simulink model "ac3_example_MMCT"  (R2023a)
settings: Solver=FixedStepDiscrete  StartTime=0.0  StopTime=3  FixedStep=Ts  RelTol=1e-3  EnableMultiTasking=on
PreLoadFcn:
  | Ts = 2e-6;
undefined symbols (not defined in the file): DiscIntNeverNeededParam
libraries: simulink_extras x7, spsCurrentMeasurementLib x3, spsVoltageMeasurementLib x3, spsDrivesPrivateModels x2, spsStairGeneratorLib x2, spsThreePhaseSourceLib x1, spsDrivesDcBusModel x1, spsSpaceVectorModulatorLib x1, eeAdaptiveController x1, slctrlblks x1, simulink x1, slpidlib x1
(part 1 of 3)
settings Model: Creator=The MathWorks, Inc.  LastModifiedBy=13372
settings SolverCC: AlgebraicLoopSolver=TrustRegion
settings DataIOCC: LimitDataPoints=on  SaveFormat=Array  SaveOutput=off  SignalLogging=off  SaveTime=off  ReturnWorkspaceOutputs=off  SignalLoggingName=sigsOut
settings OptimizationCC: ExpressionDepthLimit=2147483647  InitFltsAndDblsToZero=on  LifeSpan=inf
settings DebuggingCC: UnderspecifiedInitializationDetection=Classic  MergeDetectMultiDrivingBlocksExec=none  CheckExecutionContextPreStartOutputMsg=on  SignalResolutionControl=TryResolveAllWithWarning  MultiTaskDSMMsg=warning  MultiTaskCondExecSysMsg=none  FcnCallInpInsideContextMsg=warning  UnconnectedInputMsg=warning  UnconnectedOutputMsg=warning  UnconnectedLineMsg=warning  StateNameClashWarn=warning  SFUnexpectedBacktrackingDiag=warning  SFNoUnconditionalDefaultTransitionDiag=warning  SFExecutionAtInitializationDiag=none  ArithmeticOperatorsInVariantConditions=warning
settings HardwareCC: ProdBitPerPointer=32  ProdBitPerSizeT=32  ProdBitPerPtrDiffT=32  ProdLargestAtomicFloat=None  ProdIntDivRoundTo=Undefined  ProdEndianess=Unspecified  ProdWordSize=32  ProdHWDeviceType=32-bit Generic  TargetUnknown=on
settings ModelReferenceCC: EnableRefExpFcnMdlSchedulingChecks=on  PropagateSignalLabelsOutOfModel=off
settings SFSimCC: SimUseLocalCustomCode=off  CustomCodeUndefinedFunction=UseInterfaceOnly
settings RTWCC: RTWUseLocalCustomCode=off
settings CodeAppCC: StateflowObjectComments=on
settings GRTTargetCC: TargetLangStandard=C89/C90 (ANSI)  CombineOutputUpdateFcns=off  GRTInterface=on
settings ConfigComp: CovMetricSettings=dw  CovSaveCumulativeToWorkspaceVar=on  CovSaveSingleToWorkspaceVar=on  CovExternalEMLEnable=off  CovSFcnEnable=off
settings SimscapeCC: SimscapeNormalizeSystem=off

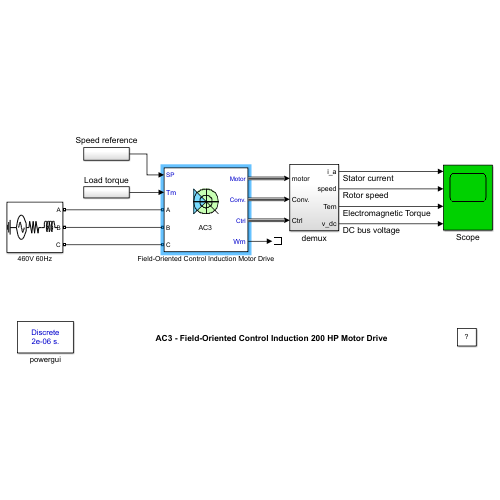
[thumbnail: Simulink's stored preview of the top-level diagram]
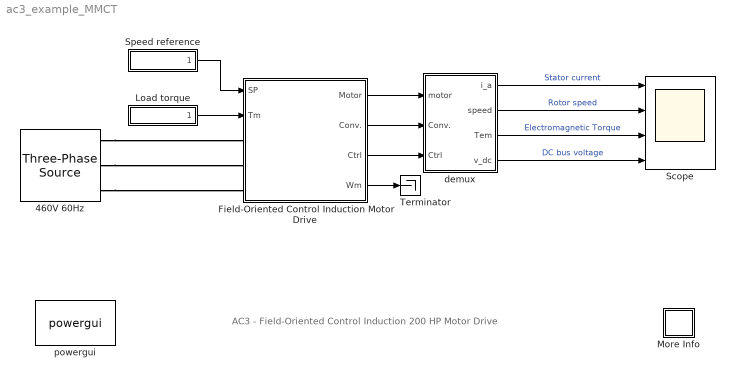
== system ac3_example_MMCT ==
  note: AC3 - Field-Oriented Control Induction 200 HP Motor Drive
  460V 60Hz : spsThreePhaseSourceLib/Three-Phase Source  InternalConnection=Yg  VoltagePhases=off  Voltage=460  PhaseAngle=0  Voltage_phases=[25e3 25e3 25e3]/sqrt(3)  PhaseAngles_phases=[0 -120 +120]  Frequency=60  NonIdealSource=on  SpecifyImpedance=off  Resistance=0.02  Inductance=0.05e-3  ShortCircuitLevel=100e6  BaseVoltage=25e3  XRratio=7  BusType=swing  Pref=0  Qref=0  Prefabc=[10e3, 10e3, 10e3]  Qrefabc=[0, 0, 0]  Qmin=-inf  Qmax=inf
  Field-Oriented Control Induction Motor Drive : Subsystem  AncestorBlock=electricdrivelib/AC drives/Field-Oriented Control Induction Motor Drive  DialogController=POWERSYS.PowerSysDialog  LoadFcn=|  mask(Field-Oriented Control Induction Motor Drive){ReferenceFrame=Rotor, IterativeDiscreteModel=Trapezoidal non iterative, Pn=149.2e3, Vn=460, fn=60, Rs=14.85e-3, Lls=0.3027e-3, Lms=10.46e-3, Rr=9.295e-3, Llr=0.3027e-3, ia=0, pha=0, ib=0, phb=0, ic=0, phc=0, J=3.1, Friction=0.08, p=2, slip=1, thdeg=0, Rsnb_rec=10e3, Csnb_rec=20e-9, Ron_rec=1e-3, Vf_rec=1.3, cap_bus=7500e-6, Rbrake=8, fbrake=4000, activationVoltage=700, shutdownVoltage=660, sourceFrequency=60, deviceType=IGBT / Diodes, Ron_inv=1e-3, Vf_inv=0.8, Vfd_inv=0.8, Tf=1e-6, Tt=2e-6, Tf_GTO=10e-6, Tt_GTO=20e-6, Rsnb_inv=5e3, Csnb_inv=inf, regulationType=Speed regulation, Acc=900, Dec=-900, kp_sc=300, ki_sc=2000, fc_sc=1000, Tsc=100e-6, Tmin=-1200, Tmax=1200, in_flux=0.73, nf=0.73, kp_fc=100, ki_fc=30, freqc_fc=16, fluxmin=-2, fluxmax=2, modulationType=SVM, h=10, kp_Id=5, ki_Id=100, kp_Iq=5, ki_Iq=100, fc_bus=50, car_freq=20000, freq_max=20000, Tvect=20e-6, zeta=0.9, Trd=0.1, bwRatio=30, kp_estimator=5000, ki_estimator=50, upperLimit=500, lowerLimit=-500, Testimator=2e-06, baseSampleTime=2e-06, outputBusMode=Multiple output buses, busLabels=off, sensorless=off, MechanicalLoad=Torque Tm, modelDetailLevel=Detailed, driveType=AC3, AverageValue=off}
      | if ~isempty(get_param(gcb,'UserData')) 
      |       UserDataToSimulinkMask(gcbh,get_param(gcb,'driveType'));  
      |       set_param(gcb, 'UserData',[]);
      |       set_param(gcb,'UserDataPersistent','off');
      | end 
      | 
      | if strcmp(get_param(gcb,'AverageValue'),'on')
      |     set_param(gcb,'modelDetailLevel','Average');
      | end
      mask prompts: ReferenceFrame "Reference frame:"; IterativeDiscreteModel "Discrete solver model:"; Pn "Power (VA):"; Vn "Voltage (Vrms):"; fn "Frequency (Hz):"; Rs "Resistance (ohm):"; Lls "Leakage inductance (H):"; Lms "Mutual inductance (H):"; Rr "Resistance (ohms):"; Llr "Leakage inductance (H):"; ia "Ia_Magnitude (A)"; pha "Ia_Phase (deg)"; ib "Ib_Magnitude (A)"; phb "Ib_Phase (deg)"; ic "Ic_Magnitude (A)"; phc "Ic_Phase (deg)"; J "Inertia (kg.m^2):"; Friction "Friction factor (N.m.s):"; p "Pole pairs:"; thdeg "Angle (deg):"; Rsnb_rec "Resistance (ohm):"; Csnb_rec "Capacitance (F):"; Ron_rec "On-state resistance (ohm):"; Vf_rec "Forward voltage (V):"; cap_bus "Capacitance (F):"; Rbrake "Resistance (ohm):"; fbrake "Chopper frequency (Hz):"; activationVoltage "Activation voltage (V):"; shutdownVoltage "Shutdown voltage (V):"; sourceFrequency "Source frequency (Hz):"; deviceType "Device type:"; Ron_inv "On-state resistance (ohm):"; Vf_inv "Main device:"; Vfd_inv "Diode:"; Tf "Fall time (s):"; Tt "Tail time (s):"; Tf_GTO "Fall time (s):"; Tt_GTO "Tail time (s):"; Rsnb_inv "Resistance (ohm):"; Csnb_inv "Capacitance (F):"; regulationType "Regulation type:"; Acc "Acceleration:"; Dec "Deceleration:"; kp_sc "Proportional gain:"; ki_sc "Integral gain:"; fc_sc "Speed cutoff frequency (Hz):"; Tsc "Speed controller sampling time (s):"; Tmin "Negative:"; Tmax "Positive:"; in_flux "Initial:"; nf "Nominal:"; kp_fc "Proportional gain:"; ki_fc "Integral gain:"; freqc_fc "Low-pass filter cutoff frequency (Hz):"; fluxmin "Negative:"; fluxmax "Positive:"; modulationType "Modulation type:"; h "Current controller hysteresis bandwidth (A):"; kp_Id "Proportional gain:"; ki_Id "Integral gain:"; kp_Iq "Proportional gain:"; ki_Iq "Integral gain:"; fc_bus "DC bus voltage sensor cutoff frequency (Hz):"; car_freq "SVM switching frequency (Hz):"; freq_max "Maximum  switching frequency (Hz):"; Tvect "Controller sampling time (s):"; zeta "Desired damping [zeta] :"; Trd "Desired response time @ 5% [Trd (sec)] :"; bwRatio "Bandwidth ratio (InnerLoop/SpeedLoop) :"; kp_estimator "Proportional gain:"; ki_estimator "Integral gain:"; upperLimit "Upper:"; lowerLimit "Lower:"; Testimator "Controller Sample Time"; baseSampleTime "Base sample time:"; outputBusMode "Output bus mode:"; busLabels "Use bus labels"; sensorless "Set sensorless"; MechanicalLoad "Mechanical input:"; modelDetailLevel "Model detail level:"; driveType "Drive type:"; AverageValue "Average value model"
      mask help: Implements a standard vector or rotor field-oriented control drive for induction motors.
      mask init:
      | [X1,X1m,X2,X2m,X3,X4,Y1,Y1m,Y2,Y2m,Y3,Y4,color1,color2,INp,OUTp,machineType,baseSampleTime] = spsDrivesMaskInit(gcb,driveType,AverageValue);
      settings: OpenFcn=sps_rtmsupport('OpenFcn',gcbh)
      settings: LibrarySourceBlock=|
      | electricdrivelib/AC drives/Field-Oriented Control
      | Induction Motor Drive
      mask Help: helpview(psbhelp)
      mask TypeOptions ReferenceFrame: Rotor | Stationary | Synchronous
      mask Callback ReferenceFrame: set_param([gcb '/Induction machine'],'ReferenceFrame',get_param(gcb,'ReferenceFrame'));
      mask TypeOptions IterativeDiscreteModel: Forward Euler | Trapezoidal non iterative
      mask Callback IterativeDiscreteModel: %set_param(gcb,'IterativeDiscreteModel',get_param([gcb '/Induction machine'],'IterativeModel'));
      mask Callback Pn: %set(gcf,'Color',[0.3,0.7,0.1])
      mask TypeOptions deviceType: GTO / Diodes | MOSFET / Diodes | IGBT / Diodes
      mask Callback deviceType:
      | set_param([gcb,'/Three-phase Inverter'],'Device',get_param(gcb,'deviceType'));
      | spsDrivesMaskController(gcb,get_param(gcb,'driveType'),get_param(gcb,'averageValue'));
      mask TypeOptions regulationType: Speed regulation | Torque regulation
      mask Callback regulationType:
      | set_param([gcb '/Speed Controller'],'SwK',get_param(gcb,'regulationType'));
      | spsDrivesMaskController(gcb,get_param(gcb,'driveType'),get_param(gcb,'averageValue'));
      mask TypeOptions modulationType: Hysteresis | SVM
      mask Callback modulationType:
      | spsDrivesMaskController(gcb,get_param(gcb,'driveType'),get_param(gcb,'averageValue'));
      | %spsDrivesSetModulation(gcb,get_param(gcb,'driveType'),get_param(gcb,'averageValue'));
      mask TypeOptions outputBusMode: Multiple output buses | Single output bus
      mask Callback sensorless:
      | %spsDrivesSetSensorless(gcb,get_param(gcb,'driveType'),get_param(gcb,'sensorless'));
      | spsDrivesMaskController(gcb,get_param(gcb,'driveType'),get_param(gcb,'averageValue'));
      | %spsDrivesSetSensorless(gcb,get_param(gcb,'driveType'),get_param(gcb,'sensorless'));
      | %spsDrivesMaskController(gcb,get_param(gcb,'driveType'),get_param(gcb,'averageValue'));
      mask TypeOptions MechanicalLoad: Torque Tm | Speed w | Mechanical rotational port
      mask Callback MechanicalLoad: spsDrivesMaskController(gcb,get_param(gcb,'driveType'),get_param(gcb,'averageValue'));
      mask TypeOptions modelDetailLevel: Detailed | Average
      mask Callback modelDetailLevel:
      | if strcmp(get_param(gcb,'modelDetailLevel'),'Average')
      |    set_param(gcb,'AverageValue','on');
      |    spsDrivesMaskController(gcb,get_param(gcb,'driveType'),1);
      | else
      |    set_param(gcb,'AverageValue','off');
      |    spsDrivesMaskController(gcb,get_param(gcb,'driveType'),0);
      | end
      mask TypeOptions driveType: AC3
      mask DialogControl Container7 Prompt: Asynchronous Machine
      mask DialogControl Container22 Prompt: Electrical parameters
      mask DialogControl Container24 Prompt: Nominal values
      mask DialogControl Container27 Prompt: Equivalent circuit values
      mask DialogControl Container25 Prompt: Main winding stator
      mask DialogControl Container21 Prompt: Main winding rotor
      mask DialogControl Container34 Prompt: Initial currents
      mask DialogControl Container23 Prompt: Mechanical parameters
      mask DialogControl Container36 Prompt: Initial  values
      mask DialogControl Container10 Prompt: Converters and DC bus
      mask DialogControl Container28 Prompt: Rectifier
      mask DialogControl Container39 Prompt: Snubbers
      mask DialogControl Container40 Prompt: Diodes
      mask DialogControl Container30 Prompt: DC bus
      mask DialogControl Container31 Prompt: Braking chopper
      mask DialogControl Container32 Prompt: Inverter
      mask DialogControl Container41 Prompt: Switches
      mask DialogControl Forwardvoltages Prompt: Forward voltages (V)
      mask DialogControl Turnoff Prompt: Turn-off characteristics
      mask DialogControl InvSnubbers Prompt: Snubbers
      mask DialogControl Container12 Prompt: Controller
      mask DialogControl Control5 Prompt: Schematic
      mask DialogControl Control5 Callback:
      | openfig('ac3.fig','invisible');
      | movegui(gcf,'northwest');
      | set(gcf,'Visible','on');
      mask DialogControl SpeedController Prompt: Speed controller
      mask DialogControl Speedramp Prompt: Speed ramps (rpm/s)
      mask DialogControl PIregulator Prompt: PI regulator
      mask DialogControl Container46 Prompt: Torque output limits (N.m)
      mask DialogControl Container37 Prompt: Machine flux (Wb)
      mask DialogControl FieldOrientedControl Prompt: Field oriented control
      mask DialogControl FluxRegulator Prompt: Flux controller
      mask DialogControl Container50 Prompt: Flux output limits (Wb)
      mask DialogControl d_axiscurrentregulator Prompt: d-axis current regulator
      mask DialogControl q_axiscurrentregulator Prompt: q-axis current regulator
      mask DialogControl autoTuningCtrlbtn Prompt: Hide Autotuning Control
      mask DialogControl autoTuningCtrlbtn Callback: spsDrivesAutotuningCbak(gcb,'visibility',get_param(gcb,'driveType'));
      mask DialogControl autoTuningContainer Prompt: Autotuning of PI loops
      mask DialogControl Control7 Prompt: Enter speed loop specifications
      mask DialogControl Calculate Prompt: Calculate PI regulators gains
      mask DialogControl Calculate Callback: spsDrivesAutotuningCbak(gcb,'PICalculator',get_param(gcb,'driveType'));
      mask DialogControl sensorlessTab Prompt: Sensorless
      mask DialogControl Container59 Prompt: Estimator controller parameters
      mask DialogControl Container61 Prompt: Output limits
      mask DialogControl Container56 Prompt: Parameters file options
      mask DialogControl Control3 Prompt: Load
      mask DialogControl Control3 Callback: loadValues(gcb,get_param(gcb,'driveType'));
      mask DialogControl Control4 Prompt: Save
      mask DialogControl Control4 Callback: saveValues(gcb,get_param(gcb,'driveType'));
      mask Display:
      | patch([X1 X1m],[Y1 Y1m],color1);
      | patch(X3,Y3,color2);
      | plot([X1 X1m X2 X2m X3 X4],[Y1 Y1m Y2 Y2m Y3 Y4]);
      | text(0.5,0.3,'AC3','HorizontalAlignment','center')
      | HaveSPSMec = (strcmp(MechanicalLoad,'Torque Tm') || strcmp(MechanicalLoad,'Speed w'));
      | color('blue');
      | if (HaveSPSMec==1 && strcmp(outputBusMode,'Multiple output buses'))
      |     port_label('input',2,INp)
      |     port_label('output',4,OUTp)
      | end
      | if (HaveSPSMec==1 && strcmp(outputBusMode,'Single output bus'))
      |     port_label('input',2,INp)
      |     port_label('output',2,OUTp)
      | end
  Load torque : Subsystem
  More Info : Subsystem
      settings: OpenFcn=showdemo(bdroot(gcb))
      mask Display: disp('?')
  Scope : Scope  NumInputPorts=4
  Speed reference : Subsystem
  Terminator : Terminator
  demux : Subsystem
  powergui : spspowerguiLib/powergui  Priority=2  SimulationMode=Discrete  SampleTime=Ts  frequency=60  Iterations=50  frequencyindice=60  Pbase=100e6  ErrMax=1e-4  UnitsV=kV  UnitsW=MW  buscounter=0  FunctionMessages=off  echomessages=off  EnableUseOfTLC=off  CurrentSourceSwitches=off  DisableSnubberDevices=off  DisableRonSwitches=off  DisableVfSwitches=off  DisplayEquations=off  AutomaticDiscreteSolvers=off  SolverType=Tustin/Backward Euler (TBE)  Interpol=off  ExternalGateDelay=off  methode=off  Ts=0  x0status=blocks  SPID=off  SwTol=0  HookPort=off  NonlinearTolerance=1e-4  nMaxIteration=100  ContinueOnMaxIteration=off  RestoreLinks=warning  ResistiveCurrentMeasurement=off  Frange=[0:2:500]  Ylog=off  Xlog=on  ShowGrid=off  save=off  variable=ZData  structure=simout  ZoomFFT=on  StartTime=0.05  cycles=7  DisplayStyle=1  fundamental=60  FreqAxis=off  MaxFrequency=20000  frequencyindicesteady=1  RmsSteady=1  display=off
  wires:
  demux/1(i_a) -> Scope/1  "Stator current"
  demux/2(speed) -> Scope/2  "Rotor speed"
  demux/3(Tem) -> Scope/3  "Electromagnetic Torque"
  demux/4(v_dc) -> Scope/4  "DC bus voltage"
  Field-Oriented Control Induction Motor Drive/1(Motor) -> demux/1(motor)
  Field-Oriented Control Induction Motor Drive/2(Conv.) -> demux/2(Conv.)
  Field-Oriented Control Induction Motor Drive/3(Ctrl) -> demux/3(Ctrl)
  Speed reference/1(" ") -> Field-Oriented Control Induction Motor Drive/1(SP)
  Load torque/1(" ") -> Field-Oriented Control Induction Motor Drive/2(Tm)
  Field-Oriented Control Induction Motor Drive/4(Wm) -> Terminator/1
  connections:
  460V 60Hz/RConn1 -- Field-Oriented Control Induction Motor Drive/LConn1
  460V 60Hz/RConn2 -- Field-Oriented Control Induction Motor Drive/LConn2
  460V 60Hz/RConn3 -- Field-Oriented Control Induction Motor Drive/LConn3

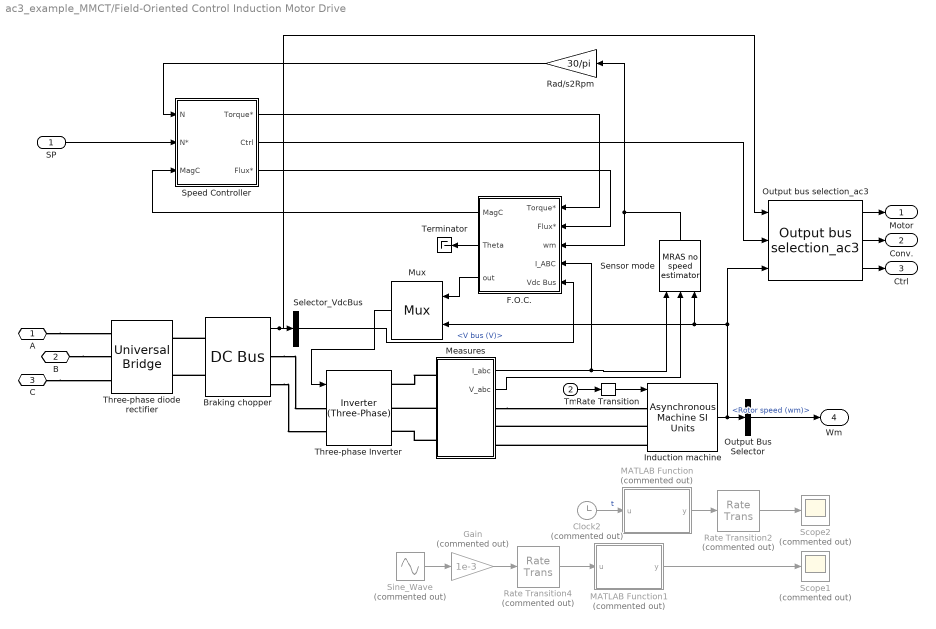
== system ac3_example_MMCT/Field-Oriented Control Induction Motor Drive ==
  SP : Inport
  Tm : Inport  Port=2
  Braking chopper : spsDrivesDcBusModel/DC Bus   busType=Capacitive (generic)  Ts=baseSampleTime  capacitance=cap_bus  inductance=0  Setx0=off  InitialVoltage=600  Rbrake=Rbrake  frequency=fbrake  activationVoltage=activationVoltage  shutdownVoltage=shutdownVoltage
  Clock2 : Clock  Commented=on
      settings: Decimation=3
  F.O.C. : Subsystem  AncestorBlock=spsFieldOrientedControllerLib/Field-Oriented Controller  DialogController=POWERSYS.PowerSysDialog  Variant=on  VariantControlMode=label  LabelModeActiveChoice=Detailed_SVM  mask(Field-Oriented Controller){detailLevel=Detailed, modulationType=SVM, kp=kp_fc, ki=ki_fc, fc=freqc_fc, csat=[fluxmin,fluxmax], Tvect=Tvect, Ts=baseSampleTime, h=h, freq_max=freq_max, fc_bus=fc_bus, car_freq=car_freq, kp_Id=kp_Id, ki_Id=ki_Id, kp_Iq=kp_Iq, ki_Iq=ki_Iq, Rr=Rr, Llr=Llr, Lm=Lms, p=p, in_flux=in_flux}
      mask prompts: detailLevel "Model detail level"; modulationType "Modulation type"; kp "Proportional gain"; ki "Integral gain"; fc "Low-pass filter cutoff frequency (Hz)"; csat "Controller output flux saturation (Wb) [Negative, Positive]"; Tvect "Vector control sampling time (s)"; Ts "Base sample time (s)"; h "Current regulator hysteresis bandwidth (A)"; freq_max "Maximum inverter frequency (Hz)"; fc_bus "DC bus voltage sensor cutoff frequency (Hz)"; car_freq "SVM switching frequency (Hz)"; kp_Id "Proportional gain"; ki_Id "Integral gain"; kp_Iq "Proportional gain"; ki_Iq "Integral gain"; Rr "Rotor resistance Rr' (Ohms)"; Llr "Rotor leakage inductance Llr' (H)"; Lm "Mutual inductance Lm (H)"; p "Pairs of poles"; in_flux "Initial flux (Wb)"
      mask help: This block implements a field oriented controller.
      mask init:
      | Lr=Lm+Llr;
      | [X1,X1m,X2,X2m,X3,X4,Y1,Y1m,Y2,Y2m,Y3,Y4,color1,color2]=spsdrivelogo;
      | block=gcb;
      | spsDrivesFieldOrientedControllercCbak(block);
      settings: AttributesFormatString=%<BlockChoice>  LibrarySourceBlock=spsFieldOrientedControllerLib/Field-Oriented Controller  OpenFcn=sps_rtmsupport('OpenFcn',gcbh)
      mask Help: helpview(psbhelp);
      mask TypeOptions detailLevel: Detailed | Average
      mask Callback detailLevel: spsDrivesFieldOrientedControllercCbak(gcb);
      mask TypeOptions modulationType: Hysteresis | SVM
      mask Callback modulationType: spsDrivesFieldOrientedControllercCbak(gcb);
      mask DialogControl ParameterTabVar01 Prompt: Controller
      mask DialogControl Container7 Prompt: Flux controller
      mask DialogControl daxis_gbox Prompt: d-axis current regulator
      mask DialogControl qaxis_gbox Prompt: q-axis current regulator
      mask DialogControl ParameterTabVar012 Prompt: Machine
      mask Display:
      | patch([X1 X1m],[Y1 Y1m],color1);
      | patch(X3,Y3,color2);
      | plot([X1 X1m X2 X2m X3 X4],[Y1 Y1m Y2 Y2m Y3 Y4]);
      | block=gcb;
      | detailLevel = get_param(block,'detailLevel');
      | color('blue');
      | switch detailLevel
      |     case 'Detailed'
      |         port_label('output',3,'Gates');
      |     case 'Average'
      |         port_label('output',3,'sig*');
      | end
  Gain : Gain  Commented=on  Gain=1e-3
  Induction machine : spsAsynchronousMachineSIUnitsLib/Asynchronous Machine SI Units  RotorType=Squirrel-cage  PresetModel=No  MechanicalLoad=Torque Tm  ShowDetailedParameters=on  ReferenceFrame=Rotor  Units=SI  MeasurementBus=off  NominalParameters="[Pn  Vn  fn]"  VoltageRatio=1  Stator=[Rs Lls]  Rotor=[Rr Llr]  Cage1=[ 0.022 0.226/377]  Cage2=[ 0.022 0.226/377]  Lm=Lms  Mechanical="[J  Friction p]"  PolePairs=2  InitialConditions=[slip,thdeg,ia,ib,ic,pha,phb,phc]  SimulateSaturation=off  Saturation=[0 0;0 0]  LoadFlowParameters=0  TsPowergui=0  TsBlock=-1  IterativeModel=Trapezoidal non iterative  IterativeDiscreteModel=Trapezoidal non iterative  Pmec=0
      settings: AttributesFormatString=\n
  MATLAB Function : MATLAB Function  Commented=on  TreatAsAtomicUnit=on
  MATLAB Function1 : MATLAB Function  Commented=on  TreatAsAtomicUnit=on
  Measures : Subsystem
  Mux : spsDrivesPrivateModels/Mux  LabelModeActiveChoice=Detailed  detailLevel=Detailed  driveType=AC3
      settings: AttributesFormatString=%<BlockChoice>
  Output Bus Selector : BusSelector  OutputSignals=Mechanical.Rotor speed (wm)
  Output bus selection_ac3 : spsDrivesOutputSelector/Output bus selection_ac3  SystemSampleTime=-1  LabelModeActiveChoice=Multiple_output_buses  VariantActivationTime=update diagram  Latency=0  AutoFrameSizeCalculation=off
      settings: AttributesFormatString=%<BlockChoice>
  Rad/s2Rpm : Gain  Gain=30/pi  SaturateOnIntegerOverflow=on  OutDataTypeStr=Inherit: Same as input  ParamDataTypeStr=Inherit: Same as input
  Rate Transition : RateTransition  OutPortSampleTime=baseSampleTime
  Rate Transition2 : RateTransition  Commented=on
  Rate Transition4 : RateTransition  Commented=on
  Scope1 : Scope  Commented=on
  Scope2 : Scope  Commented=on
  Selector_VdcBus : BusSelector  OutputSignals=V bus (V)
  Sensor mode : spsDrivesEstimatorBlock/MRAS no speed estimator  SystemSampleTime=-1  VariantActivationTime=update diagram  Latency=0  AutoFrameSizeCalculation=off
  Sine_Wave : Sin  Commented=on  Amplitude=2  Bias=1  Frequency=20  SampleTime=0
  Speed Controller : Subsystem  AncestorBlock=|  DialogController=POWERSYS.PowerSysDialog  mask(Speed Controller (AC)){ctrlType=With flux reference output, SwK=Speed regulation, Ts=baseSampleTime, ramp=[Dec,Acc], kp=kp_sc, ki=ki_sc, fc=fc_sc, ctrl_sat=[Tmin,Tmax], Tsc=Tsc, fn=fn, p=p, nf=nf}
      | spsDrivesSpeedControllerModel/Speed Controller
      | (AC)
      mask prompts: ctrlType "Controller type"; SwK "Regulation type"; Ts "Base sample time (s)"; ramp "Speed reference ramp (rpm/s) [Deceleration, Acceleration]"; kp "Proportional gain"; ki "Integral gain"; fc "Low-pass filter cutoff frequency (Hz)"; ctrl_sat "Output torque saturation (N.m) [Negative, Positive]"; Tsc "Sample time (s)"; fn "Nominal frequency (Hz)"; p "Pairs of poles"; nf "Nominal flux (Wb)"
      mask help: This block implements a PI speed regulator for AC machines.
      mask init:
      | bs=2*30*fn/p;
      | [X1,X1m,X2,X2m,X3,X4,Y1,Y1m,Y2,Y2m,Y3,Y4,color1,color2]=spsdrivelogo;
      | block=gcb;
      | spsDrivesSpeedControllerAcCbak(block,'init');
      | switch SwK
      |     case 'Torque regulation'
      |         reg_mode=2;
      |     case 'Speed regulation'
      |         reg_mode=1;
      |     otherwise
      |         error(['Unknow regulation mode ''',SwK,'''.'])
      | end
      settings: OpenFcn=sps_rtmsupport('OpenFcn',gcbh)
      settings: LibrarySourceBlock=|
      | spsDrivesSpeedControllerModel/Speed Controller
      | (AC)
      mask Help: helpview(psbhelp);
      mask TypeOptions ctrlType: With flux reference output | Without flux reference output
      mask Callback ctrlType: spsDrivesSpeedControllerAcCbak(gcb,'maskVisibilities');
      mask TypeOptions SwK: Speed regulation | Torque regulation
      mask Callback SwK: spsDrivesSpeedControllerAcCbak(gcb,'maskVisibilities');
      mask DialogControl ParameterTabVar01 Prompt: Controller
      mask DialogControl ParameterTabVar012 Prompt: Machine
      mask Display:
      | offset=0.1;
      | patch([X1 X1m],[Y1 Y1m]-offset,color1);
      | patch(X3,Y3-offset,color2);
      | plot([X1 X1m X2 X2m X3 X4],[Y1 Y1m Y2 Y2m Y3 Y4]-offset);
      | 
      | switch SwK
      |     case 'Speed regulation'
      |         label = 'Speed';
      |     case 'Torque regulation'
      |         label = 'Torque';
      | end
      | text(0.5,0.9,label,'HorizontalAlignment','center');
  Terminator : Terminator
  Three-phase diode rectifier : spsUniversalBridgeLib/Universal Bridge  Arms=3  SnubberResistance=Rsnb_rec  SnubberCapacitance=Csnb_rec  Device=Diodes  Ron=Ron_rec  Lon=0  ForwardVoltages="[  0,  0  ]"  ForwardVoltage=Vf_rec  GTOparameters=[ 10e-6, 20e-6 ]  IGBTparameters=[ 1e-6 , 2e-6 ]  Measurements=All voltages and currents  Measurements_2=None  converterType=Rectifier
      settings: AttributesFormatString=\n
  Three-phase Inverter : spsInverterThreePhaseLib/Inverter (Three-Phase)  LabelModeActiveChoice=Detailed  detailLevel=Detailed  driveType=Field-oriented control  Ts=baseSampleTime  SnubberResistance=Rsnb_inv  SnubberCapacitance=Csnb_inv  Device=IGBT / Diodes  Ron=Ron_inv  ForwardVoltages="[  Vf_inv  Vfd_inv  ]"  GTOparameters=[Tf_GTO,Tt_GTO]  IGBTparameters="[  Tf  Tt  ]"  Measurements=All voltages and currents  converterType=Inverter  SourceFrequency=sourceFrequency  ReferenceFrame=Rotor  dqInductances=[0 0]  Inductance=0  Ls=0  Resistance=0  Flux=0  Stator_sm=0  Stator_im=[Rs Lls]  Rotor=[Rr Llr]  Lm=Lms  p=p
  A : PMIOPort  Side=Left
  B : PMIOPort  Port=2  Side=Left
  C : PMIOPort  Port=3  Side=Left
  Motor : Outport  VectorParamsAs1DForOutWhenUnconnected=off
  Conv. : Outport  Port=2  VectorParamsAs1DForOutWhenUnconnected=off
  Ctrl : Outport  Port=3  VectorParamsAs1DForOutWhenUnconnected=off
  Wm : Outport  Port=4  VectorParamsAs1DForOutWhenUnconnected=off
  wires:
  F.O.C./3(out) -> Mux/1
  Speed Controller/3(Flux*) -> F.O.C./2(Flux*)
  Speed Controller/1(Torque*) -> F.O.C./1(Torque*)
  Speed Controller/2(Ctrl) -> Output bus selection_ac3/2
  Output bus selection_ac3/3 -> Ctrl/1
  Output bus selection_ac3/2 -> Conv./1
  Output bus selection_ac3/1 -> Motor/1
  Mux/1 -> Three-phase Inverter/1
  Braking chopper/1 -> Selector_VdcBus/1, Output bus selection_ac3/1
  SP/1 -> Speed Controller/2(N*)
  Rad/s2Rpm/1 -> Speed Controller/1(N)
  F.O.C./1(MagC) -> Speed Controller/3(MagC)
  F.O.C./2(Theta) -> Terminator/1
  Measures/1(I_abc) -> Sensor mode/1, F.O.C./4(I_ABC)
  Induction machine/1 -> Output Bus Selector/1, Output bus selection_ac3/3, Sensor mode/3, Mux/2
  Output Bus Selector/1 -> Wm/1  "<Rotor speed (wm)>"
  Tm/1 -> Rate Transition/1
  Rate Transition/1 -> Induction machine/1
  Sensor mode/1 -> Rad/s2Rpm/1, F.O.C./3(wm)
  Measures/2(V_abc) -> Sensor mode/2
  Sine_Wave/1 -> Gain/1
  MATLAB Function/1(y) -> Rate Transition2/1
  Clock2/1 -> MATLAB Function/1(u)  "t"
  Rate Transition4/1 -> MATLAB Function1/1(u)
  Gain/1 -> Rate Transition4/1
  MATLAB Function1/1(y) -> Scope1/1
  Rate Transition2/1 -> Scope2/1
  Selector_VdcBus/1 -> F.O.C./5(Vdc Bus)  "<V bus (V)>"
  connections:
  Braking chopper/LConn2 -- Three-phase diode rectifier/RConn2
  Measures/LConn3 -- Three-phase Inverter/RConn3
  Braking chopper/LConn1 -- Three-phase diode rectifier/RConn1
  A/RConn1 -- Three-phase diode rectifier/LConn1
  B/RConn1 -- Three-phase diode rectifier/LConn2
  C/RConn1 -- Three-phase diode rectifier/LConn3
  Braking chopper/RConn1 -- Three-phase Inverter/LConn1
  Braking chopper/RConn2 -- Three-phase Inverter/LConn2
  Measures/LConn1 -- Three-phase Inverter/RConn1
  Measures/RConn1 -- Induction machine/LConn1
  Measures/LConn2 -- Three-phase Inverter/RConn2
  Induction machine/LConn2 -- Measures/RConn2
  Induction machine/LConn3 -- Measures/RConn3

== system ac3_example_MMCT/Load torque ==
  Stair Generator : spsStairGeneratorLib/Stair Generator  t=[0 0.5 1.5]  e=[0 792 -792]  Ts=Ts
  " " : Outport  VectorParamsAs1DForOutWhenUnconnected=off
  wires:
  Stair Generator/1 -> " "/1

== system ac3_example_MMCT/More Info ==

== system ac3_example_MMCT/Speed reference ==
  Stair Generator : spsStairGeneratorLib/Stair Generator  t=[0 1]  e=[500 0]  Ts=Ts
  " " : Outport  VectorParamsAs1DForOutWhenUnconnected=off
  wires:
  Stair Generator/1 -> " "/1

== system ac3_example_MMCT/demux ==
  note: speed reference
  motor : Inport
  Conv. : Inport  Port=2
  Ctrl : Inport  Port=3
  Bus Selector : BusSelector  OutputSignals=Stator measurements.Stator current is_a (A),Mechanical.Rotor speed (wm),Mechanical.Electromagnetic torque Te (N*m)
  Bus Selector1 : BusSelector  OutputSignals=V bus (V)
  Bus Selector2 : BusSelector  OutputSignals=Torque reference (Nm),Reference
  Gain : Gain  Gain=30/pi  SaturateOnIntegerOverflow=on  OutDataTypeStr=Inherit: Same as input  ParamDataTypeStr=Inherit: Same as input
  Mux1 : Mux  Commented=on  Inputs=2
  Mux2 : Mux  Commented=on  Inputs=2
  i_a : Outport  VectorParamsAs1DForOutWhenUnconnected=off
  speed : Outport  Port=2  VectorParamsAs1DForOutWhenUnconnected=off
  Tem : Outport  Port=3  VectorParamsAs1DForOutWhenUnconnected=off
  v_dc : Outport  Port=4  VectorParamsAs1DForOutWhenUnconnected=off
  wires:
  motor/1 -> Bus Selector/1
  Gain/1 -> speed/1
  Bus Selector/2 -> Gain/1  "<Rotor speed (wm)>"
  Bus Selector/1 -> i_a/1  "<Stator current is_a (A)>"
  Conv./1 -> Bus Selector1/1
  Bus Selector1/1 -> v_dc/1  "<V bus (V)>"
  Ctrl/1 -> Bus Selector2/1
  Bus Selector/3 -> Tem/1  "<Electromagnetic torque Te (N*m)>"

== system ac3_example_MMCT/Field-Oriented Control Induction Motor Drive/F.O.C. ==
  Torque* : Inport
  Flux* : Inport  Port=2
  wm : Inport  Port=3
  I_ABC : Inport  Port=4
  Vdc Bus : Inport  Port=5
  Average : Subsystem  VariantControl=Average
  Detailed : Subsystem  VariantControl=Detailed
  Detailed SVM : Subsystem  VariantControl=Detailed_SVM
  MagC : Outport  VectorParamsAs1DForOutWhenUnconnected=off
  Theta : Outport  Port=2  VectorParamsAs1DForOutWhenUnconnected=off
  out : Outport  Port=3  VectorParamsAs1DForOutWhenUnconnected=off

== system ac3_example_MMCT/Field-Oriented Control Induction Motor Drive/Measures ==
  Current Measurement : spsCurrentMeasurementLib/Current Measurement  Tag=PoWeRsYsTeMmEaSuReMeNt  PhasorSimulation=off  OutputType=Complex  PSBequivalent=0
      settings: AttributesFormatString=\n
  Current Measurement1 : spsCurrentMeasurementLib/Current Measurement  Tag=PoWeRsYsTeMmEaSuReMeNt  PhasorSimulation=off  OutputType=Complex  PSBequivalent=0
      settings: AttributesFormatString=\n
  Current Measurement2 : spsCurrentMeasurementLib/Current Measurement  Tag=PoWeRsYsTeMmEaSuReMeNt  PhasorSimulation=off  OutputType=Complex  PSBequivalent=0
      settings: AttributesFormatString=\n
  Mux1 : Mux  Inputs=3
  Mux2 : Mux  Inputs=3
  Voltage Measurement : spsVoltageMeasurementLib/Voltage Measurement  PhasorSimulation=off  OutputType=Complex  PSBequivalent=0
  Voltage Measurement1 : spsVoltageMeasurementLib/Voltage Measurement  PhasorSimulation=off  OutputType=Complex  PSBequivalent=0
  Voltage Measurement2 : spsVoltageMeasurementLib/Voltage Measurement  PhasorSimulation=off  OutputType=Complex  PSBequivalent=0
  Ta : PMIOPort  Side=Left
  Tb : PMIOPort  Port=2  Side=Left
  Tc : PMIOPort  Port=3  Side=Left
  Mta : PMIOPort  Port=4  Side=Right
  Mtb : PMIOPort  Port=5  Side=Right
  Mtc : PMIOPort  Port=6  Side=Right
  I_abc : Outport  VectorParamsAs1DForOutWhenUnconnected=off
  V_abc : Outport  Port=2  VectorParamsAs1DForOutWhenUnconnected=off
  wires:
  Voltage Measurement2/1 -> Mux2/3
  Voltage Measurement1/1 -> Mux2/2
  Voltage Measurement/1 -> Mux2/1
  Mux2/1 -> V_abc/1
  Current Measurement2/1 -> Mux1/3
  Current Measurement/1 -> Mux1/1
  Current Measurement1/1 -> Mux1/2
  Mux1/1 -> I_abc/1
  connections:
  Voltage Measurement1/LConn2 -- Mtc/RConn1 -- Voltage Measurement2/LConn2 -- Current Measurement2/RConn1
  Tc/RConn1 -- Current Measurement2/LConn1
  Ta/RConn1 -- Current Measurement/LConn1
  Voltage Measurement2/LConn1 -- Voltage Measurement/LConn1 -- Mta/RConn1 -- Current Measurement/RConn1
  Tb/RConn1 -- Current Measurement1/LConn1
  Voltage Measurement1/LConn1 -- Mtb/RConn1 -- Current Measurement1/RConn1 -- Voltage Measurement/LConn2

== system ac3_example_MMCT/Field-Oriented Control Induction Motor Drive/Speed Controller ==
  N : Inport
  N* : Inport  Port=2
  MagC : Inport  Port=3
  Speed Controller (AC) : Subsystem  Variant=on  VariantControlMode=label  LabelModeActiveChoice=AC345
      settings: AttributesFormatString=%<BlockChoice>
  Torque* : Outport  VectorParamsAs1DForOutWhenUnconnected=off
  Ctrl : Outport  Port=2  VectorParamsAs1DForOutWhenUnconnected=off
  Flux* : Outport  Port=3  VectorParamsAs1DForOutWhenUnconnected=off
  wires:
  N*/1 -> Speed Controller (AC)/2(N*)
  Speed Controller (AC)/1(Flux*) -> Flux*/1
  MagC/1 -> Speed Controller (AC)/3(MagC)
  N/1 -> Speed Controller (AC)/1(N)
  Speed Controller (AC)/2(Torque*) -> Torque*/1
  Speed Controller (AC)/3(Ctrl) -> Ctrl/1

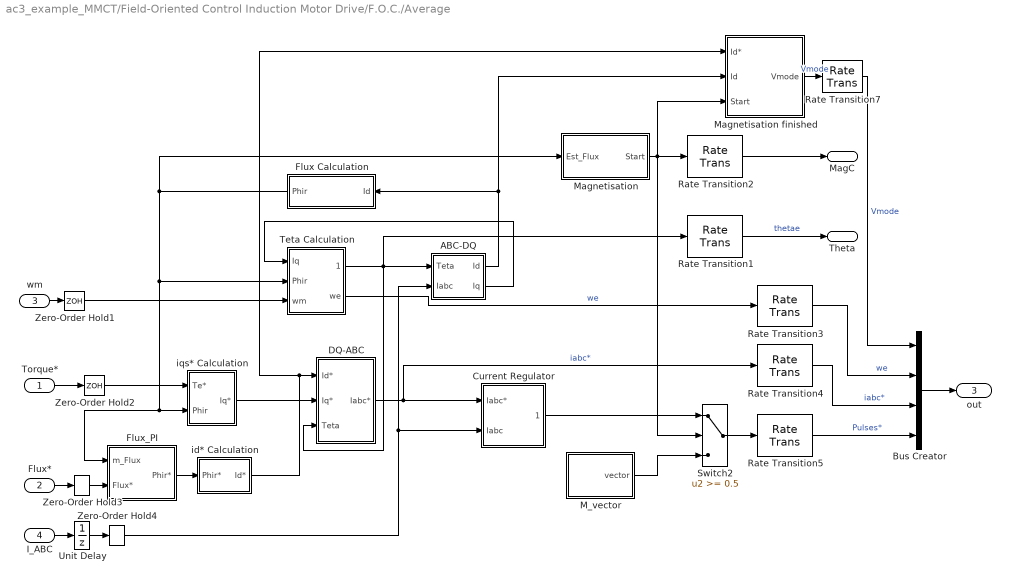
== system ac3_example_MMCT/Field-Oriented Control Induction Motor Drive/F.O.C./Average ==
  Torque* : Inport
  Flux* : Inport  Port=2
  wm : Inport  Port=3
  I_ABC : Inport  Port=4
  ABC-DQ : Subsystem
  Bus Creator : BusCreator  Inputs=4
  Current Regulator : Subsystem  TreatAsAtomicUnit=on
  DQ-ABC : Subsystem
  Flux Calculation : Subsystem  mask(Flux Calcultation){}
      mask init:
      | NF=0.44572610323020e-6;
      | DF=[1 -0.99998715486734];
  Flux_PI : Subsystem
  M_vector : Subsystem
  Magnetisation : Subsystem
  Magnetisation finished : Subsystem
  Rate Transition1 : RateTransition  OutPortSampleTime=Ts
  Rate Transition{2..5,7} (5 alike) : RateTransition
  Switch2 : Switch  Threshold=0.5  InputSameDT=off
  Teta Calculation : Subsystem
  Unit Delay : UnitDelay  SampleTime=-1  HasFrameUpgradeWarning=on
  Zero-Order Hold{1..4} (4 alike) : ZeroOrderHold  SampleTime=Tvect
  id* Calculation : Subsystem
  iqs* Calculation : Subsystem
  MagC : Outport  VectorParamsAs1DForOutWhenUnconnected=off
  Theta : Outport  Port=2  VectorParamsAs1DForOutWhenUnconnected=off
  out : Outport  Port=3  VectorParamsAs1DForOutWhenUnconnected=off
  wires:
  Unit Delay/1 -> Zero-Order Hold4/1
  Switch2/1 -> Rate Transition5/1
  M_vector/1(vector) -> Switch2/3
  Current Regulator/1(Pulses) -> Switch2/1
  Bus Creator/1 -> out/1
  DQ-ABC/1(Iabc*) -> Current Regulator/1(Iabc*), Rate Transition4/1  "iabc*"
  Rate Transition5/1 -> Bus Creator/4  "Pulses*"
  Flux_PI/1(Phir*) -> id* Calculation/1(Phir*)
  Zero-Order Hold1/1 -> Teta Calculation/3(wm)
  Zero-Order Hold4/1 -> Current Regulator/2(Iabc), ABC-DQ/2(Iabc)
  Zero-Order Hold2/1 -> iqs* Calculation/1(Te*)
  Rate Transition1/1 -> Theta/1  "thetae"
  Magnetisation/1(Start) -> Rate Transition2/1, Magnetisation finished/3(Start), Switch2/2
  Flux*/1 -> Zero-Order Hold3/1
  Torque*/1 -> Zero-Order Hold2/1
  wm/1 -> Zero-Order Hold1/1
  I_ABC/1 -> Unit Delay/1
  Teta Calculation/1(Thetae) -> Rate Transition1/1, DQ-ABC/3(Teta), ABC-DQ/1(Teta)
  id* Calculation/1(Id*) -> DQ-ABC/1(Id*), Magnetisation finished/1(Id*)
  iqs* Calculation/1(Iq*) -> DQ-ABC/2(Iq*)
  Flux Calculation/1(Phir) -> Magnetisation/1(Est_Flux), Flux_PI/1(m_Flux), iqs* Calculation/2(Phir), Teta Calculation/2(Phir)
  ABC-DQ/2(Iq) -> Teta Calculation/1(Iq)
  ABC-DQ/1(Id) -> Flux Calculation/1(Id), Magnetisation finished/2(Id)
  Rate Transition2/1 -> MagC/1
  Rate Transition3/1 -> Bus Creator/2  "we"
  Rate Transition4/1 -> Bus Creator/3  "iabc*"
  Magnetisation finished/1(Vmode) -> Rate Transition7/1  "Vmode"
  Teta Calculation/2(we) -> Rate Transition3/1  "we"
  Rate Transition7/1 -> Bus Creator/1  "Vmode"
  Zero-Order Hold3/1 -> Flux_PI/2(Flux*)

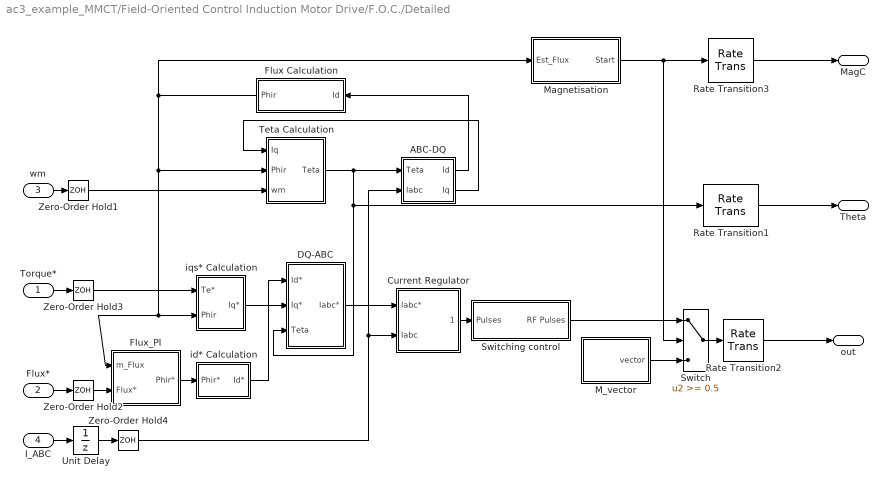
== system ac3_example_MMCT/Field-Oriented Control Induction Motor Drive/F.O.C./Detailed ==
  Torque* : Inport
  Flux* : Inport  Port=2
  wm : Inport  Port=3
  I_ABC : Inport  Port=4
  ABC-DQ : Subsystem
  Current Regulator : Subsystem
  DQ-ABC : Subsystem
  Flux Calculation : Subsystem  mask(Flux Calcultation){}
      mask init:
      | NF=0.44572610323020e-6;
      | DF=[1 -0.99998715486734];
  Flux_PI : Subsystem
  M_vector : Subsystem
  Magnetisation : Subsystem
  Rate Transition1 : RateTransition  OutPortSampleTime=Ts
  Rate Transition2 : RateTransition
  Rate Transition3 : RateTransition
  Switch : Switch  Threshold=0.5  InputSameDT=off
  Switching control : Subsystem
  Teta Calculation : Subsystem
  Unit Delay : UnitDelay  SampleTime=-1  HasFrameUpgradeWarning=on
  Zero-Order Hold{1..4} (4 alike) : ZeroOrderHold  SampleTime=Tvect
  id* Calculation : Subsystem
  iqs* Calculation : Subsystem
  MagC : Outport  VectorParamsAs1DForOutWhenUnconnected=off
  Theta : Outport  Port=2  VectorParamsAs1DForOutWhenUnconnected=off
  out : Outport  Port=3  VectorParamsAs1DForOutWhenUnconnected=off
  wires:
  Unit Delay/1 -> Zero-Order Hold4/1
  Flux_PI/1(Phir*) -> id* Calculation/1(Phir*)
  Zero-Order Hold1/1 -> Teta Calculation/3(wm)
  Zero-Order Hold4/1 -> ABC-DQ/2(Iabc), Current Regulator/2(Iabc)
  Zero-Order Hold3/1 -> iqs* Calculation/1(Te*)
  Rate Transition1/1 -> Theta/1
  Rate Transition3/1 -> MagC/1
  Rate Transition2/1 -> out/1
  M_vector/1(vector) -> Switch/3
  Magnetisation/1(Start) -> Rate Transition3/1, Switch/2
  Switch/1 -> Rate Transition2/1
  DQ-ABC/1(Iabc*) -> Current Regulator/1(Iabc*)
  Flux*/1 -> Zero-Order Hold2/1
  Torque*/1 -> Zero-Order Hold3/1
  Current Regulator/1(Pulses) -> Switching control/1(Pulses)
  wm/1 -> Zero-Order Hold1/1
  I_ABC/1 -> Unit Delay/1
  Teta Calculation/1(Teta) -> Rate Transition1/1, DQ-ABC/3(Teta), ABC-DQ/1(Teta)
  id* Calculation/1(Id*) -> DQ-ABC/1(Id*)
  iqs* Calculation/1(Iq*) -> DQ-ABC/2(Iq*)
  Flux Calculation/1(Phir) -> iqs* Calculation/2(Phir), Flux_PI/1(m_Flux), Teta Calculation/2(Phir), Magnetisation/1(Est_Flux)
  ABC-DQ/2(Iq) -> Teta Calculation/1(Iq)
  ABC-DQ/1(Id) -> Flux Calculation/1(Id)
  Switching control/1(RF Pulses) -> Switch/1
  Zero-Order Hold2/1 -> Flux_PI/2(Flux*)

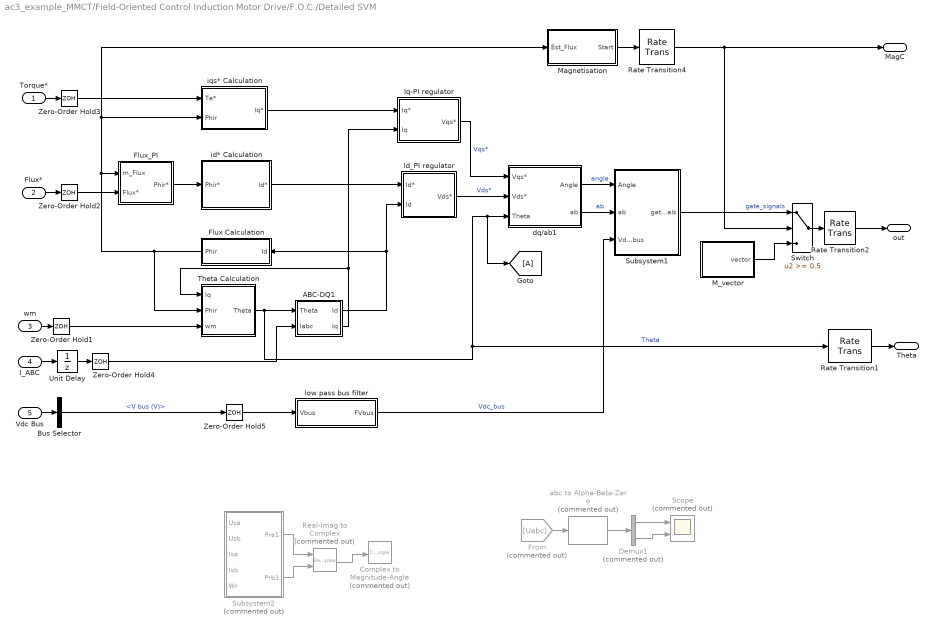
== system ac3_example_MMCT/Field-Oriented Control Induction Motor Drive/F.O.C./Detailed SVM ==
  Torque* : Inport
  Flux* : Inport  Port=2
  wm : Inport  Port=3
  I_ABC : Inport  Port=4
  Vdc Bus : Inport  Port=5
  ABC-DQ1 : Subsystem
  Bus Selector : BusSelector  OutputSignals=V bus (V)
  Complex to Magnitude-Angle : ComplexToMagnitudeAngle  Commented=on
  Demux1 : Demux  Commented=on  Outputs=2
  Flux Calculation : Subsystem  mask(Flux Calcultation){}
      mask init:
      | NF=0.44572610323020e-6;
      | DF=[1 -0.99998715486734];
  Flux_PI : Subsystem
  From : From  Commented=on  GotoTag=Uabc
  Goto : Goto
  Id_PI regulator : Subsystem
  Iq-PI regulator : Subsystem
  M_vector : Subsystem
  Magnetisation : Subsystem
  Rate Transition1 : RateTransition  OutPortSampleTime=Ts
  Rate Transition2 : RateTransition
  Rate Transition4 : RateTransition
  Real-Imag to Complex : RealImagToComplex  Commented=on
  Scope : Scope  Commented=on  NumInputPorts=2
  Subsystem1 : Subsystem
      mask Display:
      | %port_label('input',1,'{\omega_m}','texmode','on')
      | %port_label('lconn',1,'{\omega_m}','texmode','on')
      | disp('SVPWM')
      | %text(0.1,0.5,'SVM')
      | %text(0.1,0.5,'{\omega_m}','texmode','on')
      | %plot([0 1],[0 1]);
  Subsystem2 : Subsystem  Commented=on  mask{Lm=0, Lr=0, Ls=0, Sigma=0, tao=0}
      mask DialogControl ParameterGroupVar Prompt: 参数
  Switch : Switch  Threshold=0.5  InputSameDT=off
  Theta Calculation : Subsystem
  Unit Delay : UnitDelay  SampleTime=-1  HasFrameUpgradeWarning=on
  Zero-Order Hold{1..5} (5 alike) : ZeroOrderHold  SampleTime=Tvect
  abc to Alpha-Beta-Zero : spsabctoAlphaBetaZeroLib/abc to Alpha-Beta-Zero  Commented=on
  dq/ab1 : Subsystem
      mask Display:
      | %text(0.1,0.5,'SVM')
      | text(0.2,0.6,'dq')
      | text(0.7,0.4,'\alpha\beta','texmode','on')
      | plot([0 1],[0 1]);
  id* Calculation : Subsystem
  iqs* Calculation : Subsystem
  low pass bus filter : Subsystem
  MagC : Outport  VectorParamsAs1DForOutWhenUnconnected=off
  Theta : Outport  Port=2  VectorParamsAs1DForOutWhenUnconnected=off
  out : Outport  Port=3  VectorParamsAs1DForOutWhenUnconnected=off
  wires:
  Unit Delay/1 -> Zero-Order Hold4/1
  Flux_PI/1(Phir*) -> id* Calculation/1(Phir*)
  Zero-Order Hold1/1 -> Theta Calculation/3(wm)
  Zero-Order Hold3/1 -> iqs* Calculation/1(Te*)
  Rate Transition1/1 -> Theta/1
  Magnetisation/1(Start) -> Rate Transition4/1
  Rate Transition2/1 -> out/1
  M_vector/1(vector) -> Switch/3
  Switch/1 -> Rate Transition2/1
  Flux*/1 -> Zero-Order Hold2/1
  Torque*/1 -> Zero-Order Hold3/1
  wm/1 -> Zero-Order Hold1/1
  I_ABC/1 -> Unit Delay/1
  Flux Calculation/1(Phir) -> Theta Calculation/2(Phir), Magnetisation/1(Est_Flux), iqs* Calculation/2(Phir), Flux_PI/1(m_Flux)
  ABC-DQ1/2(Iq) -> Iq-PI regulator/2(Iq), Theta Calculation/1(Iq)
  Zero-Order Hold2/1 -> Flux_PI/2(Flux*)
  Zero-Order Hold5/1 -> low pass bus filter/1(Vbus)
  Vdc Bus/1 -> Bus Selector/1
  Bus Selector/1 -> Zero-Order Hold5/1  "<V bus (V)>"
  ABC-DQ1/1(Id) -> Id_PI regulator/2(Id), Flux Calculation/1(Id)
  iqs* Calculation/1(Iq*) -> Iq-PI regulator/1(Iq*)
  id* Calculation/1(Id*) -> Id_PI regulator/1(Id*)
  Zero-Order Hold4/1 -> ABC-DQ1/2(Iabc)
  Theta Calculation/1(Theta) -> ABC-DQ1/1(Theta), Rate Transition1/1, Goto/1, dq/ab1/3(Theta)  "Theta"
  Subsystem1/1(gate_signals) -> Switch/1  "gate_signals"
  Iq-PI regulator/1(Vqs*) -> dq/ab1/1(Vqs*)  "Vqs*"
  Id_PI regulator/1(Vds*) -> dq/ab1/2(Vds*)  "Vds*"
  dq/ab1/1(Angle) -> Subsystem1/1(Angle)  "angle"
  dq/ab1/2(ab) -> Subsystem1/2(ab)  "ab"
  low pass bus filter/1(FVbus) -> Subsystem1/3(Vdc_bus)  "Vdc_bus"
  Rate Transition4/1 -> MagC/1, Switch/2
  Subsystem2/1(Pra1) -> Real-Imag to Complex/1
  Subsystem2/2(Prb1) -> Real-Imag to Complex/2
  Real-Imag to Complex/1 -> Complex to Magnitude-Angle/1
  From/1 -> abc to Alpha-Beta-Zero/1
  abc to Alpha-Beta-Zero/1 -> Demux1/1
  Demux1/1 -> Scope/1
  Demux1/2 -> Scope/2

== system ac3_example_MMCT/Field-Oriented Control Induction Motor Drive/Speed Controller/Speed Controller (AC) ==
  N : Inport
  N* : Inport  Port=2
  MagC : Inport  Port=3
  AC345 : Subsystem  VariantControl=AC345
  AC678 : Subsystem  VariantControl=AC678
  Flux* : Outport  VectorParamsAs1DForOutWhenUnconnected=off
  Torque* : Outport  Port=2  VectorParamsAs1DForOutWhenUnconnected=off
  Ctrl : Outport  Port=3  VectorParamsAs1DForOutWhenUnconnected=off

== system ac3_example_MMCT/Field-Oriented Control Induction Motor Drive/F.O.C./Average/ABC-DQ ==
  Teta : Inport
  Iabc : Inport  Port=2
  Fcn : Fcn  Expr=sin(u)
  Fcn1 : Fcn  Expr=cos(u)
  Gain : Gain  Gain=2/3  SaturateOnIntegerOverflow=on  OutDataTypeStr=Inherit: Same as input  ParamDataTypeStr=Inherit: Same as input
  Gain1 : Gain  Gain=2/3  SaturateOnIntegerOverflow=on  OutDataTypeStr=Inherit: Same as input  ParamDataTypeStr=Inherit: Same as input
  Mux : Mux  Inputs=[1 1 3]
  id : Fcn  Expr=u[1]*u[3]+(1.7320508*u[2]-u[1])*u[4]*0.5+(-u[1]-1.7320508*u[2])*u[5]*0.5
  iq : Fcn  Expr=-u[2]*u[3]+(u[2]+1.7320508*u[1])*u[4]*0.5+(u[2]-1.7320508*u[1])*u[5]*0.5
  Id : Outport  InitialOutput=0  VectorParamsAs1DForOutWhenUnconnected=off
  Iq : Outport  Port=2  InitialOutput=0  VectorParamsAs1DForOutWhenUnconnected=off
  wires:
  Gain1/1 -> Iq/1
  Gain/1 -> Id/1
  id/1 -> Gain/1
  iq/1 -> Gain1/1
  Iabc/1 -> Mux/3
  Mux/1 -> id/1, iq/1
  Teta/1 -> Fcn/1, Fcn1/1
  Fcn1/1 -> Mux/1
  Fcn/1 -> Mux/2

== system ac3_example_MMCT/Field-Oriented Control Induction Motor Drive/F.O.C./Average/Current Regulator ==
  Iabc* : Inport
  Iabc : Inport  Port=2
  Demux1 : Demux  Outputs=3
      settings: DisplayOption=none
  Demux2 : Demux  Outputs=3
      settings: DisplayOption=none
  Mux1 : Mux  Inputs=2
  Relay : Relay  OnSwitchValue=0  OffSwitchValue=-0
  Relay1 : Relay  OnSwitchValue=0  OffSwitchValue=-0
  Relay2 : Relay  OnSwitchValue=0  OffSwitchValue=-0
  Sum : Sum  Inputs=-+  InputSameDT=on  SaturateOnIntegerOverflow=on  OutDataTypeStr=Inherit: Same as first input
  Sum1 : Sum  Inputs=-+  InputSameDT=on  SaturateOnIntegerOverflow=on  OutDataTypeStr=Inherit: Same as first input
  Sum2 : Sum  Inputs=-+  InputSameDT=on  SaturateOnIntegerOverflow=on  OutDataTypeStr=Inherit: Same as first input
  Sum3 : Sum  Inputs=+-
  Sum4 : Sum  Inputs=+-
  Pulses : Outport  InitialOutput=0  VectorParamsAs1DForOutWhenUnconnected=off
  wires:
  Sum4/1 -> Mux1/2
  Sum3/1 -> Mux1/1
  Relay2/1 -> Sum4/2
  Relay1/1 -> Sum4/1, Sum3/2
  Relay/1 -> Sum3/1
  Iabc*/1 -> Demux2/1
  Demux2/1 -> Sum/2
  Demux2/2 -> Sum1/2
  Demux2/3 -> Sum2/2
  Demux1/3 -> Sum2/1
  Sum2/1 -> Relay2/1
  Iabc/1 -> Demux1/1
  Mux1/1 -> Pulses/1
  Demux1/2 -> Sum1/1
  Demux1/1 -> Sum/1
  Sum1/1 -> Relay1/1
  Sum/1 -> Relay/1

== system ac3_example_MMCT/Field-Oriented Control Induction Motor Drive/F.O.C./Average/DQ-ABC ==
  Id* : Inport
  Iq* : Inport  Port=2
  Teta : Inport  Port=3
  Fcn : Fcn  Expr=sin(u)
  Fcn1 : Fcn  Expr=cos(u)
  Gain2 : Gain  SaturateOnIntegerOverflow=on  OutDataTypeStr=Inherit: Same as input  ParamDataTypeStr=Inherit: Same as input
  Gain3 : Gain  SaturateOnIntegerOverflow=on  OutDataTypeStr=Inherit: Same as input  ParamDataTypeStr=Inherit: Same as input
  Gain4 : Gain  SaturateOnIntegerOverflow=on  OutDataTypeStr=Inherit: Same as input  ParamDataTypeStr=Inherit: Same as input
  Mux : Mux
  Mux2 : Mux  Inputs=3
  ia : Fcn  Expr=-u[3]*u[2] + u[4]*u[1]
  ib : Fcn  Expr=(-u[1]+1.7320508*u[2])*u[4]*0.5+(u[2]+1.7320508*u[1])*u[3]*0.5
  ic : Sum  Inputs=--  InputSameDT=on  SaturateOnIntegerOverflow=on  OutDataTypeStr=Inherit: Same as first input
  Iabc* : Outport  InitialOutput=0  VectorParamsAs1DForOutWhenUnconnected=off
  wires:
  ib/1 -> ic/1, Gain3/1
  ia/1 -> ic/2, Gain2/1
  Gain2/1 -> Mux2/1
  Gain4/1 -> Mux2/3
  ic/1 -> Gain4/1
  Gain3/1 -> Mux2/2
  Id*/1 -> Mux/4
  Iq*/1 -> Mux/3
  Teta/1 -> Fcn/1, Fcn1/1
  Mux/1 -> ia/1, ib/1
  Mux2/1 -> Iabc*/1
  Fcn1/1 -> Mux/1
  Fcn/1 -> Mux/2

== system ac3_example_MMCT/Field-Oriented Control Induction Motor Drive/F.O.C./Average/Flux Calculation ==
  note: Phir = Lm *Id / (1 +Tr .s)
  Id : Inport
  Discrete Transfer Fcn1 : DiscreteTransferFcn  Numerator=[1-exp(-(Rr/(Lr))*Tvect)]  Denominator=[1 -exp(-(Rr/(Lr))*Tvect)]  SampleTime=Tvect
  Lm : Gain  Gain=Lm  SaturateOnIntegerOverflow=on  OutDataTypeStr=Inherit: Same as input  ParamDataTypeStr=Inherit: Same as input
  Phir : Outport  VectorParamsAs1DForOutWhenUnconnected=off
  wires:
  Lm/1 -> Discrete Transfer Fcn1/1
  Id/1 -> Lm/1
  Discrete Transfer Fcn1/1 -> Phir/1

== system ac3_example_MMCT/Field-Oriented Control Induction Motor Drive/F.O.C./Average/Flux_PI ==
  m_Flux : Inport
  Flux* : Inport  Port=2
  Discrete Transfer Fcn1 : DiscreteTransferFcn  Numerator=[1-exp(-(2*pi*fc)*Tvect)]  Denominator=[1 -exp(-(2*pi*fc)*Tvect)]  SampleTime=Tvect
  Discrete-Time Integrator : DiscreteIntegrator  IntegratorMethod=Integration: Trapezoidal  SampleTime=Tvect  LimitOutput=on  UpperSaturationLimit=csat(2)  LowerSaturationLimit=csat(1)  ICPrevOutput=DiscIntNeverNeededParam  ICPrevScaledInput=DiscIntNeverNeededParam
  Ki1 : Gain  Gain=ki  SaturateOnIntegerOverflow=on  OutDataTypeStr=Inherit: Same as input  ParamDataTypeStr=Inherit: Same as input
  Kp : Gain  Gain=kp  SaturateOnIntegerOverflow=on  OutDataTypeStr=Inherit: Same as input  ParamDataTypeStr=Inherit: Same as input
  Saturation : Saturate  UpperLimit=csat(2)  LowerLimit=csat(1)
  Sum : Sum  Inputs=|+-  SaturateOnIntegerOverflow=on
  Sum1 : Sum  Inputs=|++  SaturateOnIntegerOverflow=on
  Phir* : Outport  VectorParamsAs1DForOutWhenUnconnected=off
  wires:
  Sum/1 -> Kp/1, Ki1/1
  Discrete-Time Integrator/1 -> Sum1/1
  Kp/1 -> Sum1/2
  Sum1/1 -> Saturation/1
  Discrete Transfer Fcn1/1 -> Sum/2
  Flux*/1 -> Sum/1
  Saturation/1 -> Phir*/1
  m_Flux/1 -> Discrete Transfer Fcn1/1
  Ki1/1 -> Discrete-Time Integrator/1

== system ac3_example_MMCT/Field-Oriented Control Induction Motor Drive/F.O.C./Average/M_vector ==
  Constant1 : Constant  Value=[0 0]
  Constant3 : Constant  Value=[1 -1]
  Pulse Generator1 : DiscretePulseGenerator  Period=8  PulseWidth=2  SampleTime=Tvect
  Switch1 : Switch  Threshold=0.5  InputSameDT=off
  Zero-Order Hold8 : ZeroOrderHold  SampleTime=Tvect
  vector : Outport  VectorParamsAs1DForOutWhenUnconnected=off
  wires:
  Switch1/1 -> vector/1
  Zero-Order Hold8/1 -> Switch1/2
  Pulse Generator1/1 -> Zero-Order Hold8/1
  Constant1/1 -> Switch1/3
  Constant3/1 -> Switch1/1

== system ac3_example_MMCT/Field-Oriented Control Induction Motor Drive/F.O.C./Average/Magnetisation ==
  Est_Flux : Inport
  Constant : Constant  Value=in_flux
  Constant1 : Constant  Value=0
  Data Type Conversion5 : DataTypeConversion
  Relational Operator : RelationalOperator  InputSameDT=off
  S-R Flip-Flop : simulink_extras/Flip Flops/S-R Flip-Flop  initial_condition=0
  Terminator : Terminator
  Zero-Order Hold5 : ZeroOrderHold  SampleTime=Tvect
  Start : Outport  VectorParamsAs1DForOutWhenUnconnected=off
  wires:
  Zero-Order Hold5/1 -> Relational Operator/2
  S-R Flip-Flop/2 -> Terminator/1
  S-R Flip-Flop/1 -> Start/1
  Constant1/1 -> Data Type Conversion5/1
  Constant/1 -> Zero-Order Hold5/1
  Relational Operator/1 -> S-R Flip-Flop/1
  Est_Flux/1 -> Relational Operator/1
  Data Type Conversion5/1 -> S-R Flip-Flop/2

== system ac3_example_MMCT/Field-Oriented Control Induction Motor Drive/F.O.C./Average/Magnetisation finished ==
  note: Vmode = 1 when magnetisation (voltage mode)
      | Ensure that id = id* before switch to current mode
  Id* : Inport
  Id : Inport  Port=2
  Start : Inport  Port=3
  Constant1 : Constant  Value=0
  Data Type Conversion5 : DataTypeConversion
  Hit Crossing : HitCross
  Logical Operator : Logic  AllPortsSameDT=off  OutDataTypeStr=boolean
  S-R Flip-Flop : simulink_extras/Flip Flops/S-R Flip-Flop  initial_condition=0
  Sum : Sum  Inputs=+-
  Terminator : Terminator
  Vmode : Outport  VectorParamsAs1DForOutWhenUnconnected=off
  wires:
  S-R Flip-Flop/1 -> Terminator/1
  Id/1 -> Sum/2
  Start/1 -> Logical Operator/2
  Id*/1 -> Sum/1
  Sum/1 -> Hit Crossing/1
  Hit Crossing/1 -> Logical Operator/1
  Data Type Conversion5/1 -> S-R Flip-Flop/2
  Constant1/1 -> Data Type Conversion5/1
  Logical Operator/1 -> S-R Flip-Flop/1
  S-R Flip-Flop/2 -> Vmode/1  "Vmode"
